simulink model "trajectory_planning_dev_py"  (R2018b)
settings: Solver=ode2  StartTime=0.0  StopTime=inf  FixedStep=0.002  RelTol=1e-3  EnableMultiTasking=on
model workspace (MAT data in the model file):
  m = 1000
settings Model: DataDictionary=trajectory_planning_dev_py.sldd  PauseTimes=6.42  Creator=wischnewski  LastModifiedBy=ge34qer
settings DataIOCC: SaveOutput=off  SignalLogging=off  DSMLogging=off  SaveTime=off
settings OptimizationCC: StrengthReduction=on  PassReuseOutputArgsAs=Individual arguments  OptimizeBlockOrder=speed  OptimizationPriority=Speed  OptimizationCustomize=off
settings DebuggingCC: UnderspecifiedInitializationDetection=Classic  MergeDetectMultiDrivingBlocksExec=none  ParameterTunabilityLossMsg=error
settings ModelReferenceCC: PropagateSignalLabelsOutOfModel=off
settings SFSimCC: MATLABDynamicMemAlloc=off
settings RTWCC: SystemTargetFile=ert.tlc  GenCodeOnly=on  PackageGeneratedCodeAndArtifacts=on  PackageName=trajectory_planning_dev_py  TemplateMakefile=ert_default_tmf  IncludeHyperlinkInReport=on  TargetLang=C++
settings CodeAppCC: ForceParamTrailComments=on  IgnoreCustomStorageClasses=off  MaxIdLength=64  OperatorAnnotations=on  SimulinkDataObjDesc=on  SFDataObjDesc=on  InsertBlockDesc=on
settings ERTTargetCC: TargetLangStandard=C++03 (ISO)  GenerateSampleERTMain=on  MultiInstanceERTCode=on  CodeInterfacePackaging=Reusable function  SupportContinuousTime=on  SupportVariableSizeSignals=on  GenerateAllocFcn=on  RootIOFormat=Part of model data structure  RTWCAPIParams=on  ERTCustomFileTemplate=example_file_process.tlc

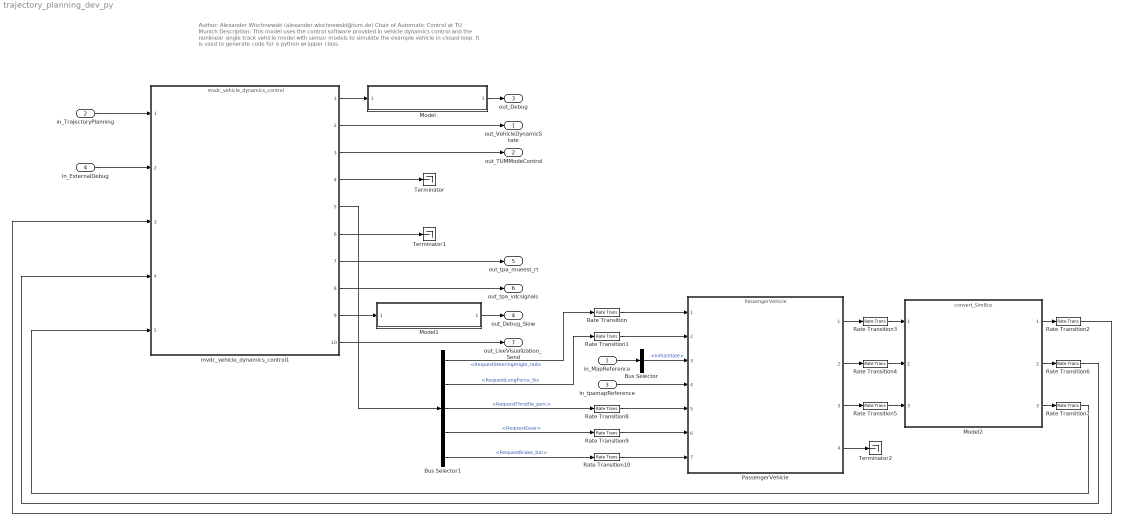
== system trajectory_planning_dev_py ==
  note: Author: Alexander Wischnewski (alexander.wischnewski@tum.de)
      | Chair of Automatic Control at TU Munich
      |
      | Description: This model uses the control software provided in vehicle dynamics control and the nonlinear single track vehicle model
      | with sensor models to simulate the example vehicle in closed loop. It is used to generate code for a python wrapper class.
  in_MapReference : Inport  OutDataTypeStr=Bus: MapReference
  in_TrajectoryPlanning : Inport  Port=2  OutDataTypeStr=Bus: TrajectoryPlanning
  in_tpamapReference : Inport  Port=3  OutDataTypeStr=Bus: tpamapReference
  in_ExternalDebug : Inport  Port=4  OutDataTypeStr=Bus: ExternalDebug
  Bus Selector : BusSelector  OutputSignals=InitialState
  Bus Selector1 : BusSelector  OutputSignals=RequestSteeringAngle_rad,RequestLongForce_N,RequestThrottle_perc,RequestGear,RequestBrake_bar
  Model : ModelReference  ModelNameDialog=debug_conversion_debug.slx  SimulationMode=Normal  ModelReferenceVersion=1.8
  Model1 : ModelReference  ModelNameDialog=debug_conversion_debug_slow.slx  SimulationMode=Normal  ModelReferenceVersion=1.8
  Model2 : ModelReference  ModelNameDialog=convert_SimBus.slx  SimulationMode=Normal  ModelReferenceVersion=1.821
  PassengerVehicle : ModelReference  ModelNameDialog=PassengerVehicle  SimulationMode=Normal  ModelReferenceVersion=1.992
  Rate Transition{,1..10} (11 alike) : RateTransition
  Terminator : Terminator
  Terminator1 : Terminator
  Terminator2 : Terminator
  mvdc_vehicle_dynamics_control1 : ModelReference  ModelNameDialog=mvdc_vehicle_dynamics_control  SimulationMode=Normal  ModelReferenceVersion=1.797
  out_VehicleDynamicState : Outport  OutDataTypeStr=Bus: VehicleDynamicState
  out_TUMModeControl : Outport  Port=2  OutDataTypeStr=Bus: TUMModeControl
  out_Debug : Outport  Port=3
  out_Debug_Slow : Outport  Port=4
  out_tpa_mueest_rt : Outport  Port=5  OutDataTypeStr=Bus: mvdc_tpa_mueest_rt_Send
  out_tpa_vdcsignals : Outport  Port=6  OutDataTypeStr=Bus: mvdc_tpa_vdcsignals_Send
  out_LiveVisualization_Send : Outport  Port=7  OutDataTypeStr=Bus: LiveVisualization  PortDimensions=1  BusOutputAsStruct=on
  wires:
  mvdc_vehicle_dynamics_control1/7 -> out_tpa_mueest_rt/1
  mvdc_vehicle_dynamics_control1/8 -> out_tpa_vdcsignals/1
  PassengerVehicle/1 -> Rate Transition3/1
  PassengerVehicle/2 -> Rate Transition4/1
  PassengerVehicle/3 -> Rate Transition5/1
  Bus Selector1/1 -> Rate Transition/1  "<RequestSteeringAngle_rad>"
  Bus Selector1/2 -> Rate Transition1/1  "<RequestLongForce_N>"
  PassengerVehicle/4 -> Terminator2/1
  Rate Transition2/1 -> mvdc_vehicle_dynamics_control1/3
  Rate Transition6/1 -> mvdc_vehicle_dynamics_control1/4
  Rate Transition7/1 -> mvdc_vehicle_dynamics_control1/5
  Bus Selector/1 -> PassengerVehicle/3  "<InitialState>"
  Rate Transition/1 -> PassengerVehicle/1
  Rate Transition1/1 -> PassengerVehicle/2
  in_MapReference/1 -> Bus Selector/1
  in_TrajectoryPlanning/1 -> mvdc_vehicle_dynamics_control1/1
  mvdc_vehicle_dynamics_control1/2 -> out_VehicleDynamicState/1
  mvdc_vehicle_dynamics_control1/3 -> out_TUMModeControl/1
  Model/1 -> out_Debug/1
  mvdc_vehicle_dynamics_control1/1 -> Model/1
  mvdc_vehicle_dynamics_control1/9 -> Model1/1
  Model1/1 -> out_Debug_Slow/1
  in_tpamapReference/1 -> PassengerVehicle/4
  Rate Transition3/1 -> Model2/1
  Rate Transition4/1 -> Model2/2
  Rate Transition5/1 -> Model2/3
  Model2/1 -> Rate Transition2/1
  Model2/2 -> Rate Transition6/1
  Model2/3 -> Rate Transition7/1
  Bus Selector1/3 -> Rate Transition8/1  "<RequestThrottle_perc>"
  mvdc_vehicle_dynamics_control1/4 -> Terminator/1
  mvdc_vehicle_dynamics_control1/6 -> Terminator1/1
  mvdc_vehicle_dynamics_control1/10 -> out_LiveVisualization_Send/1
  mvdc_vehicle_dynamics_control1/5 -> Bus Selector1/1
  in_ExternalDebug/1 -> mvdc_vehicle_dynamics_control1/2
  Bus Selector1/4 -> Rate Transition9/1  "<RequestGear>"
  Bus Selector1/5 -> Rate Transition10/1  "<RequestBrake_bar>"
  Rate Transition10/1 -> PassengerVehicle/7
  Rate Transition9/1 -> PassengerVehicle/6
  Rate Transition8/1 -> PassengerVehicle/5
